simulink model "lab2c"  (R2020a)
settings: Solver=ode3  StartTime=0.0  StopTime=inf  FixedStep=dt  RelTol=1e-3  EnableMultiTasking=on
undefined symbols (not defined in the file): dt, Kp, tau, tStart, tWait, xFinal
libraries: lab2Library x3
settings Model: SimulationMode=external  ExtModeTrigDuration=100  Creator=Sal  LastModifiedBy=crsmyth
settings SolverCC: PositivePriorityOrder=on  AutoInsertRateTranBlk=on
settings DataIOCC: SaveOperatingPoint=on  SaveFormat=StructureWithTime  ReturnWorkspaceOutputs=off
settings OptimizationCC: EnhancedBackFolding=on  PassReuseOutputArgsAs=Individual arguments  ZeroExternalMemoryAtStartup=off  ZeroInternalMemoryAtStartup=off  MaxStackSize=64  OptimizeBlockOrder=speed  DifferentSizesBufferReuse=on  OptimizationCustomize=off  EfficientTunableParamExpr=on
settings DebuggingCC: ParameterTunabilityLossMsg=error
settings HardwareCC: ProdBitPerPointer=32  ProdBitPerSizeT=32  ProdBitPerPtrDiffT=32  ProdLargestAtomicInteger=Long  ProdLargestAtomicFloat=Double  ProdWordSize=32  ProdHWDeviceType=ARM Compatible->ARM Cortex
settings SFSimCC: MATLABDynamicMemAlloc=off
settings RTWCC: SystemTargetFile=ert.tlc  HardwareBoard=BeagleBone Blue  TemplateMakefile=ert_default_tmf  Toolchain=GNU GCC BeagleBone Blue
settings CodeAppCC: ForceParamTrailComments=on  IgnoreCustomStorageClasses=off  OperatorAnnotations=on  SimulinkDataObjDesc=on  SFDataObjDesc=on  InsertBlockDesc=on
settings ERTTargetCC: MatFileLogging=on  SupportContinuousTime=on  SupportVariableSizeSignals=on

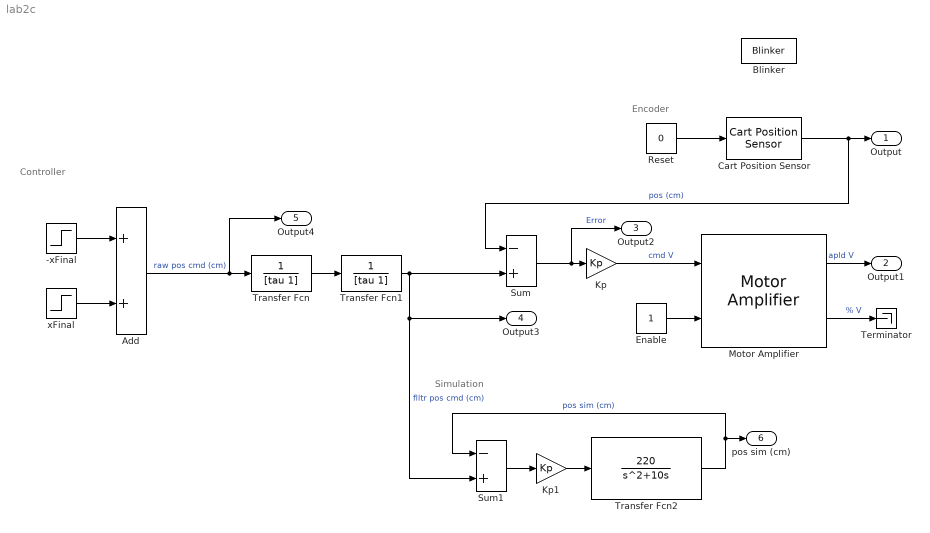
== system lab2c ==
  note: Encoder
  note: Controller
  note: Simulation
  -xFinal : Step  Time=tStart+tWait  After=-xFinal  SampleTime=0
  Add : Sum
  Blinker : lab2Library/Blinker  T=1
  Cart Position Sensor : lab2Library/Cart Position Sensor  ppr=ppr  rE=rEnc  T=dt
  Enable : Constant
  Kp : Gain  Gain=Kp
  Kp1 : Gain  Gain=Kp
  Motor Amplifier : lab2Library/Motor Amplifier  vin=6.1
  Reset : Constant  Value=0
  Sum : Sum  Inputs=-+
  Sum1 : Sum  Inputs=-+
  Terminator : Terminator
  Transfer Fcn : TransferFcn  Denominator=[tau 1]
  Transfer Fcn1 : TransferFcn  Denominator=[tau 1]
  Transfer Fcn2 : TransferFcn  Numerator=[220]  Denominator=[1 10 0]
  xFinal : Step  Time=tStart  After=xFinal  SampleTime=0
  Output : Outport
  Output1 : Outport  Port=2
  Output2 : Outport  Port=3
  Output3 : Outport  Port=4
  Output4 : Outport  Port=5
  pos sim (cm) : Outport  Port=6  SignalName=pos sim (cm)
  wires:
  Reset/1 -> Cart Position Sensor/1
  Cart Position Sensor/1 -> Sum/1, Output/1  "pos (cm)"
  Enable/1 -> Motor Amplifier/2
  Kp/1 -> Motor Amplifier/1  "cmd V"
  Motor Amplifier/1 -> Output1/1  "apld V"
  Motor Amplifier/2 -> Terminator/1  "% V"
  Sum/1 -> Output2/1, Kp/1  "Error"
  -xFinal/1 -> Add/1
  xFinal/1 -> Add/2
  Add/1 -> Output4/1, Transfer Fcn/1  "raw pos cmd (cm)"
  Transfer Fcn/1 -> Transfer Fcn1/1
  Transfer Fcn1/1 -> Sum1/2, Output3/1, Sum/2  "flltr pos cmd (cm)"
  Sum1/1 -> Kp1/1
  Kp1/1 -> Transfer Fcn2/1
  Transfer Fcn2/1 -> pos sim (cm)/1, Sum1/1  "pos sim (cm)"
